simulink model "controller2"  (R2014b)
settings: Solver=ode45  StartTime=0.0  StopTime=25  RelTol=1e-3
values from neighbouring files (symbols this model uses):
  A = [X_u + a * X_wdot * Z_u   X_w + a * X_wdot * Z_w   X_q + a * X_wdot * (u_0 + Z_q)   -g * (cos(theta_0) + a * X_wdot * sin(theta_0)) 0 ... (first row only)    [f.m]
  B = [a * X_wdot * Z_d_e + X_d_e  a * X_wdot * Z_d_T + X_d_T  -(X_u + a * X_wdot * Z_u)  -(X_w + a * X_wdot * Z_w)  -(X_q + a * X_wdot * (u_0 + Z_q)) ... (first row only)    [f.m]
  C = [1 0 0 0 0 ... (first row only)    [f.m]
  D = [0 0 0 0 0 ... (first row only)    [f.m]
settings Model: Creator=hess  LastModifiedBy=karasinski
settings DataIOCC: SignalLoggingSaveFormat=ModelDataLogs
settings OptimizationCC: ExpressionDepthLimit=2147483647
settings DebuggingCC: UnderspecifiedInitializationDetection=Classic  MergeDetectMultiDrivingBlocksExec=none  FcnCallInpInsideContextMsg=UseLocalSettings  StateNameClashWarn=warning
settings GRTTargetCC: CombineOutputUpdateFcns=off  GRTInterface=on

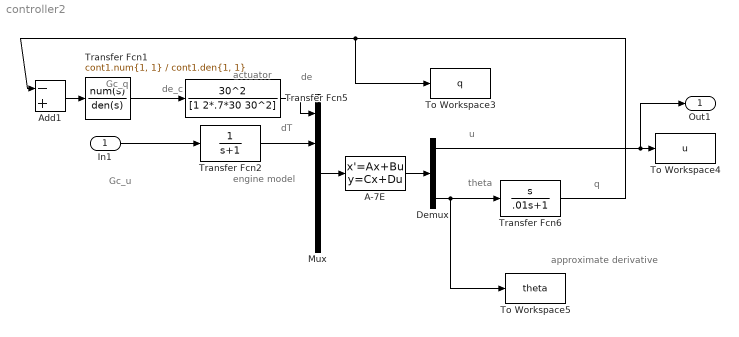
== system controller2 ==
  note: Gc_q
  note: Gc_u
  note: engine model
  note: actuator
  note: de
  note: dT
  note: q
  note: theta
  note: u
  note: de_c
  note: approximate derivative
  In1 : Inport
  A-7E : StateSpace  A=A  B=B  C=C  D=D  X0=[0 0 0 0 0]
  Add1 : Sum  Inputs=-+
  Demux : Demux  Outputs=3
  Mux : Mux  Inputs=5
  To Workspace3 : ToWorkspace  VariableName=q  SampleTime=-1
  To Workspace4 : ToWorkspace  VariableName=u  SampleTime=-1
  To Workspace5 : ToWorkspace  VariableName=theta  SampleTime=-1
  Transfer Fcn1 : TransferFcn  Numerator=cont1.num{1, 1}  Denominator=cont1.den{1, 1}
  Transfer Fcn2 : TransferFcn  Numerator=1  Denominator=[1 1]
  Transfer Fcn5 : TransferFcn  Numerator=30^2  Denominator=[1 2*.7*30 30^2]
  Transfer Fcn6 : TransferFcn  Numerator=[1 0]  Denominator=[.01 1]
  Out1 : Outport
  wires:
  A-7E/1 -> Demux/1
  Mux/1 -> A-7E/1
  Demux/3 -> To Workspace5/1, Transfer Fcn6/1
  Transfer Fcn2/1 -> Mux/2
  Demux/1 -> Out1/1, To Workspace4/1
  In1/1 -> Transfer Fcn2/1
  Transfer Fcn1/1 -> Transfer Fcn5/1
  Add1/1 -> Transfer Fcn1/1
  Transfer Fcn6/1 -> To Workspace3/1, Add1/1
  Transfer Fcn5/1 -> Mux/1
